simulink model "homework4_1_version2013b"  (R2013b)
settings: Solver=ode45  StartTime=0.0  StopTime=30.0  FixedStep=0.001  RelTol=1e-3
values from neighbouring files (symbols this model uses):
  A = [0 1;0 -b/m]    [ScriptHomework4_1.m]    (also in homework4script.m)
  Aw = 0    [ScriptHomework4_1.m]    (also in homework4script.m = [0 1; -omega^2 0])
  B = [0;1/m]    [ScriptHomework4_1.m]    (also in homework4script.m)
  b = 1/185    (= 0.00540540540541)    [ScriptHomework4_1.m]    (also in homework4script.m = 3)
  C = [1 0]    [ScriptHomework4_1.m]    (also in homework4script.m)
  Cw = 1    [ScriptHomework4_1.m]    (also in homework4script.m = [1 0])
  k = acker(A,B,[-a -a])    [ScriptHomework4_1.m]    (also in homework4script.m)
  kr = k(1)    [ScriptHomework4_1.m]
  L = L(1:end-1)    [ScriptHomework4_1.m]    (also in homework4script.m = acker(Asd',Csd',pole)')
  Lw = L(end)    [ScriptHomework4_1.m]
  m = 1/185    (= 0.00540540540541)    [ScriptHomework4_1.m]    (also in homework4script.m = 1)
  omega = 1    [ScriptHomework4_1.m]    (also in homework4script.m)
  swD = 1    [ScriptHomework4_1.m]    (also in homework4script.m = 3)
  swN = 0    [ScriptHomework4_1.m]    (also in homework4script.m)
  T = 0.01    [ScriptHomework4_1.m]
libraries: simulink x1
settings Model: Creator=milos  LastModifiedBy=milos
settings DataIOCC: LimitDataPoints=off  SaveFormat=StructureWithTime
settings DebuggingCC: UnderspecifiedInitializationDetection=Simplified  MergeDetectMultiDrivingBlocksExec=error  SolverPrmCheckMsg=none  FrameProcessingCompatibilityMsg=error
settings HardwareCC: ProdBitPerPointer=64  ProdLargestAtomicFloat=Float  ProdIntDivRoundTo=Zero  ProdEndianess=LittleEndian  ProdHWDeviceType=Specified
settings ModelReferenceCC: PropagateSignalLabelsOutOfModel=on
settings GRTTargetCC: CodeReplacementLibrary=C89/C90 (ANSI)

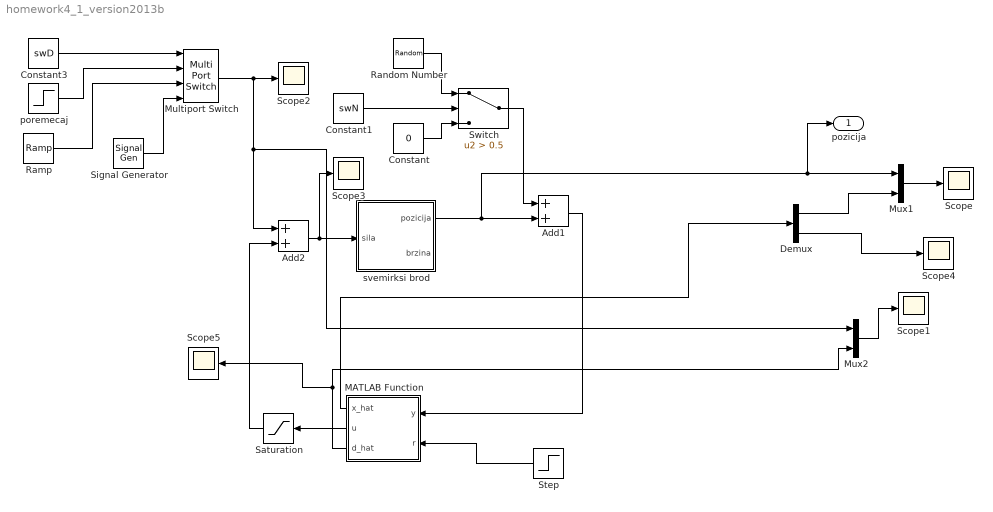
== system homework4_1_version2013b ==
  Add1 : Sum
  Add2 : Sum
  Constant : Constant  Value=0
  Constant1 : Constant  Value=swN
  Constant3 : Constant  Value=swD
  Demux : Demux  Outputs=2
  MATLAB Function : MATLAB Function  TreatAsAtomicUnit=on
      settings: PermitHierarchicalResolution=ParametersOnly
  Multiport Switch : MultiPortSwitch
  Mux1 : Mux  Inputs=2
  Mux2 : Mux  Inputs=2
  Ramp : simulink/Sources/Ramp  slope=1  start=0  X0=0
  Random Number : RandomNumber  Variance=0.01
  Saturation : Saturate  UpperLimit=1  LowerLimit=-1
  Scope{,1..5} (6 alike) : Scope
      Scope settings: TimeRange=auto  MaxDataPoints=5000  SaveToWorkspace=off  SaveName=ScopeData  YMin=-13.22485  YMax=119.02366  SampleTime=-1
      Scope1 settings: TimeRange=auto  MaxDataPoints=5000  SaveToWorkspace=off  YMin=-0.37523  YMax=3.37704  SampleTime=-1
      Scope2 settings: TimeRange=auto  MaxDataPoints=5000  SaveToWorkspace=off  SaveName=ScopeData2  YMin=-2.5  YMax=2.5  SampleTime=-1
      Scope3 settings: TimeRange=auto  MaxDataPoints=5000  SaveToWorkspace=off  SaveName=ScopeData3  YMin=-0.04033  YMax=0.0639  SampleTime=-1
      Scope4 settings: TimeRange=auto  MaxDataPoints=5000  SaveToWorkspace=off  YMin=-6.97309  YMax=41.70109  SampleTime=-1
      Scope5 settings: TimeRange=auto  MaxDataPoints=5000  SaveToWorkspace=off  SaveName=ScopeData2  YMin=-0.01252  YMax=0.11267  SampleTime=-1
  Signal Generator : SignalGenerator  Amplitude=2  Frequency=omega  Units=rad/sec
  Step : Step  After=100  SampleTime=0
  Switch : Switch  Criteria=u2 > Threshold  Threshold=0.5
  poremecaj : Step  Time=20  After=0.1  SampleTime=0
  svemirksi brod : Subsystem
  pozicija : Outport
  wires:
  Mux1/1 -> Scope/1
  Random Number/1 -> Switch/1
  Constant/1 -> Switch/3
  Constant1/1 -> Switch/2
  Switch/1 -> Add1/1
  svemirksi brod/1(pozicija) -> Add1/2, pozicija/1, Mux1/1
  Add2/1 -> Scope3/1, svemirksi brod/1(sila)
  poremecaj/1 -> Multiport Switch/2
  Ramp/1 -> Multiport Switch/3
  Constant3/1 -> Multiport Switch/1
  Multiport Switch/1 -> Scope2/1, Mux2/1, Add2/1
  Signal Generator/1 -> Multiport Switch/4
  Mux2/1 -> Scope1/1
  Add1/1 -> MATLAB Function/1(y)
  Step/1 -> MATLAB Function/2(r)
  Saturation/1 -> Add2/2
  MATLAB Function/1(x_hat) -> Demux/1
  Demux/1 -> Mux1/2
  Demux/2 -> Scope4/1
  MATLAB Function/3(d_hat) -> Scope5/1, Mux2/2
  MATLAB Function/2(u) -> Saturation/1

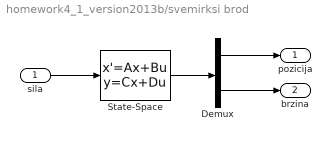
== system homework4_1_version2013b/svemirksi brod ==
  sila : Inport
  Demux : Demux  Outputs=2
  State-Space : StateSpace  A=[0 1;0 -b/m]  B=[0;1/m]  C=[1 0; 0 1]  D=[0;0]  X0=[0;0]
  pozicija : Outport
  brzina : Outport  Port=2
  wires:
  State-Space/1 -> Demux/1
  sila/1 -> State-Space/1
  Demux/1 -> pozicija/1
  Demux/2 -> brzina/1

== matlab function homework4_1_version2013b/MATLAB Function ==
  settings: updateMethod=DISCRETE  sampleTime=T
  data: y input; x_hat output; r input; u output; d_hat output; C parameter; Aw parameter; Lw parameter; Cw parameter; T parameter; A parameter; B parameter; L parameter; kr parameter; k parameter
function [x_hat,u,d_hat] = fcn(y,r,C, Aw, Lw, Cw, T, A, B, L, kr, k)

persistent  x_hat_p;
persistent w_hat_p;
if isempty(x_hat_p) || isempty(w_hat_p)
    x_hat_p=[0;0];
    w_hat_p=0;
end
d_hat=Cw*w_hat_p;
u=-k*x_hat_p+kr*r-d_hat;
if u>1
    u=1;
elseif u<-1
    u=-1;
end

x_hat=x_hat_p+T*(A*x_hat_p+B*(u+d_hat)+L*(y-C*x_hat_p));
w_hat_p=w_hat_p+T*(Aw*w_hat_p+Lw*(y-C*x_hat_p));
x_hat_p=x_hat;

end
